simulink model "acev"  (R2020a)
settings: Solver=VariableStepAuto  StartTime=0.0  StopTime=10.0  RelTol=1e-3
undefined symbols (not defined in the file): DiscIntNeverNeededParam
libraries: simrfV2junction1 x11, powerlib x7, simulink x3, simrfV2elements x2, electricdrivelib x1, powerlib_meascontrol x1
settings Model: Creator=Asish Nayak  LastModifiedBy=Asish Nayak

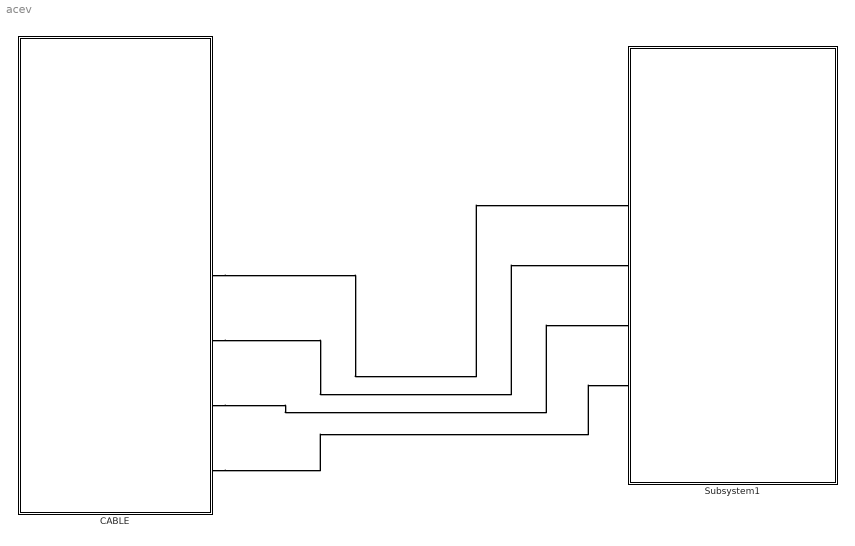
== system acev ==
  CABLE : Subsystem
  Subsystem1 : Subsystem
  connections:
  CABLE/RConn4 -- Subsystem1/LConn3
  CABLE/RConn5 -- Subsystem1/LConn4
  CABLE/RConn6 -- Subsystem1/LConn5
  CABLE/RConn7 -- Subsystem1/LConn6

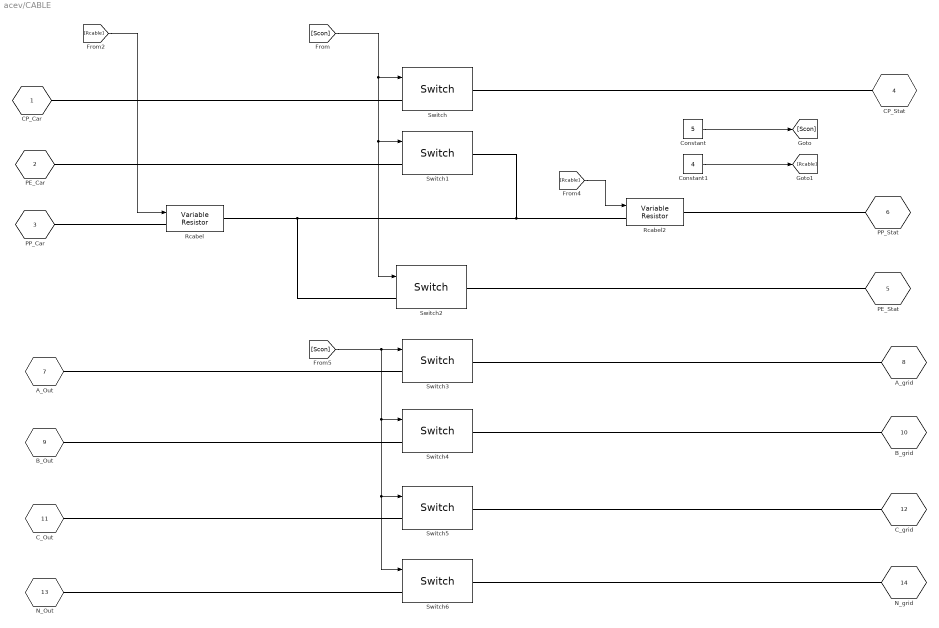
== system acev/CABLE ==
  Constant : Constant  Value=5
  Constant1 : Constant  Value=4
  Rcabel : simrfV2elements/Variable Resistor  classname=varresistor  hasNoise=on
      settings: SourceProductBaseCode=RB
  Rcabel2 : simrfV2elements/Variable Resistor  classname=varresistor  hasNoise=on
      settings: SourceProductBaseCode=RB
  Switch{,1..6} (7 alike) : simrfV2junction1/Switch  classname=switch  Ron=10 Ohm  Roff=1e6 Ohm  Vthres=0 V
      settings: SourceProductBaseCode=RB
  CP_Car : PMIOPort  Side=Left
  PE_Car : PMIOPort  Port=2  Side=Left
  PP_Car : PMIOPort  Port=3  Side=Left
  CP_Stat : PMIOPort  Port=4  Side=Right
  PE_Stat : PMIOPort  Port=5  Side=Right
  PP_Stat : PMIOPort  Port=6  Side=Right
  A_Out : PMIOPort  Port=7  Side=Left
  A_grid : PMIOPort  Port=8  Side=Right
  B_Out : PMIOPort  Port=9  Side=Left
  B_grid : PMIOPort  Port=10  Side=Right
  C_Out : PMIOPort  Port=11  Side=Left
  C_grid : PMIOPort  Port=12  Side=Right
  N_Out : PMIOPort  Port=13  Side=Left
  N_grid : PMIOPort  Port=14  Side=Right
  wires:
  Constant/1 -> [Scon]
  [Scon] -> Switch2/1, Switch1/1, Switch/1
  Constant1/1 -> [Rcable]
  [Rcable] -> Rcabel/1
  [Rcable] -> Rcabel2/1
  [Scon] -> Switch6/1, Switch5/1, Switch4/1, Switch3/1
  connections:
  CP_Car/RConn1 -- Switch/LConn1
  Switch1/LConn1 -- PE_Car/RConn1
  CP_Stat/RConn1 -- Switch/RConn1
  Rcabel/LConn1 -- PP_Car/RConn1
  Switch1/RConn1 -- Rcabel2/LConn1 -- Switch2/LConn1 -- Rcabel/RConn1
  PP_Stat/RConn1 -- Rcabel2/RConn1
  Switch2/RConn1 -- PE_Stat/RConn1
  N_Out/RConn1 -- Switch6/LConn1
  A_grid/RConn1 -- Switch3/RConn1
  C_Out/RConn1 -- Switch5/LConn1
  N_grid/RConn1 -- Switch6/RConn1
  C_grid/RConn1 -- Switch5/RConn1
  B_grid/RConn1 -- Switch4/RConn1
  A_Out/RConn1 -- Switch3/LConn1
  B_Out/RConn1 -- Switch4/LConn1

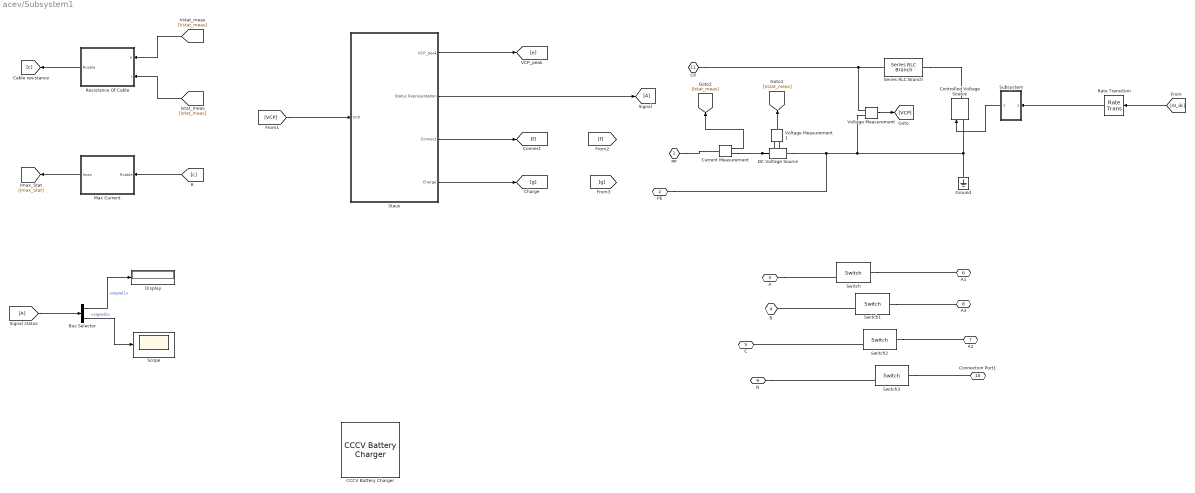
== system acev/Subsystem1 ==
  Bus Selector : BusSelector  OutputSignals=signal1,signal2
  CCCV Battery Charger : electricdrivelib/Extra Sources/CCCV Battery Charger  Preset=Custom specifications  P_nom=1500  s_type=3-phases AC (delta)  n_connect=off  eff_volt=208  in_freq=60  in_I_ripple=10  in_I_freq=1000  EFF_en=on  EFF_val=[0.627 0.803 0.855 0.871 0.872 0.864]  EFF_fu=[0.063 0.177 0.293 0.483 0.674 0.914]  THD_en=on  I_THD_val=[0.327 0.394 0.394 0.351 0.289 0.265]  I_THD_fu=[0.056 0.136 0.194 0.303 0.555 0.916]  H_DIST_rt=[0.199 1.297 0.328 0.029 0.416 0.200]  H_DIST_fr=[3 5 7 9 11 13]  PF_en=on  PF_val=[0.316 0.532 0.662 0.731 0.780 0.792]  PF_fu=[0.067 0.230 0.445 0.625 0.794 0.919]  Out_mode=Constant Current - Constant Voltage (CCCV)  DynInT=on  I_cst=10  V_cst=138  ABS_en=off  V_abs=142  ABS_end=Time based  ABS_time=3600  ABS_i=40  ripple=0.5  swF=1000  overshoot=1  stable_t=5  VoltComp=on  V_comp=-0.18  nom_temp=20
      settings: SourceProductBaseCode=PS
  Controlled Voltage Source : powerlib/Electrical Sources/Controlled Voltage Source  Initialize=off  Source_Type=DC  Amplitude=0  Phase=0  Frequency=0  Measurements=Voltage
  Current Measurement : powerlib/Measurements/Current Measurement  PhasorSimulation=off  OutputType=Complex  PSBequivalent=0
  DC Voltage Source : powerlib/Electrical Sources/DC Voltage Source  Amplitude=100  Measurements=None
  Display : Display
  Ground : powerlib/Elements/Ground  LConnTagsString=a
  Max Current : MATLAB Function  TreatAsAtomicUnit=on
  Rate Transition : RateTransition  InitialCondition=0.0  OutPortSampleTime=Tdc
  Resistance Of Cable : MATLAB Function  TreatAsAtomicUnit=on
  Scope : Scope
  Series RLC Branch : powerlib/Elements/Series RLC Branch  LConnTagsString=__new0  RConnTagsString=__new0  BranchType=R  Resistance=1000  Inductance=1e-3  SetiL0=off  InitialCurrent=0  Capacitance=1e-6  Setx0=off  InitialVoltage=0  Measurements=None
  Staus : Subsystem
  Subsystem : Subsystem
  Switch{,1..3} (4 alike) : simrfV2junction1/Switch  classname=switch  Ron=10 Ohm  Roff=1e6 Ohm  Vthres=0 V
      settings: SourceProductBaseCode=RB
  Voltage Measurement : powerlib/Measurements/Voltage Measurement  PhasorSimulation=off  OutputType=Complex  PSBequivalent=0
  Voltage Measurement1 : powerlib/Measurements/Voltage Measurement  PhasorSimulation=off  OutputType=Complex  PSBequivalent=0
  PP : PMIOPort  Side=Left
  PE : PMIOPort  Port=2  Side=Left
  A : PMIOPort  Port=3  Side=Left
  B : PMIOPort  Port=4  Side=Left
  C : PMIOPort  Port=5  Side=Left
  A1 : PMIOPort  Port=6  Side=Right
  A2 : PMIOPort  Port=7  Side=Right
  A3 : PMIOPort  Port=8  Side=Right
  N : PMIOPort  Port=9  Side=Left
  Connection Port1 : PMIOPort  Port=10  Side=Right
  CP : PMIOPort  Port=11  Side=Left
  wires:
  [SI_dc] -> Rate Transition/1
  Subsystem/1(Output) -> Controlled Voltage Source/1
  Rate Transition/1 -> Subsystem/1(Input)
  Voltage Measurement/1 -> [VCP]
  Voltage Measurement1/1 -> [Vstat_meas]
  Current Measurement/1 -> [Istat_meas]
  Bus Selector/2 -> Scope/1  "<signal2>"
  Bus Selector/1 -> Display/1  "<signal1>"
  Staus/4(Charge) -> [g]
  Staus/3(Connect) -> [f]
  Staus/1(VCP_peak) -> [e]
  [c] -> Max Current/1(Rcable)
  Staus/2(Status Representation) -> [A]
  Max Current/1(Imax) -> [Imax_Stat]
  [VCP] -> Staus/1(VCP)
  [A] -> Bus Selector/1
  [Istat_meas] -> Resistance Of Cable/2(I)
  Resistance Of Cable/1(Rcable) -> [c]
  [Vstat_meas] -> Resistance Of Cable/1(V)
  connections:
  Series RLC Branch/RConn1 -- Controlled Voltage Source/RConn1
  Voltage Measurement/LConn1 -- Series RLC Branch/LConn1 -- CP/RConn1
  Ground/LConn1 -- PE/RConn1 -- Voltage Measurement1/LConn2 -- DC Voltage Source/LConn1 -- Voltage Measurement/LConn2 -- Controlled Voltage Source/LConn1
  Current Measurement/RConn1 -- Voltage Measurement1/LConn1 -- DC Voltage Source/RConn1
  PP/RConn1 -- Current Measurement/LConn1
  A/RConn1 -- Switch/LConn1
  Switch/RConn1 -- A1/RConn1
  Switch1/LConn1 -- B/RConn1
  Switch1/RConn1 -- A3/RConn1
  Switch2/LConn1 -- C/RConn1
  Switch2/RConn1 -- A2/RConn1
  N/RConn1 -- Switch3/LConn1
  Switch3/RConn1 -- Connection Port1/RConn1

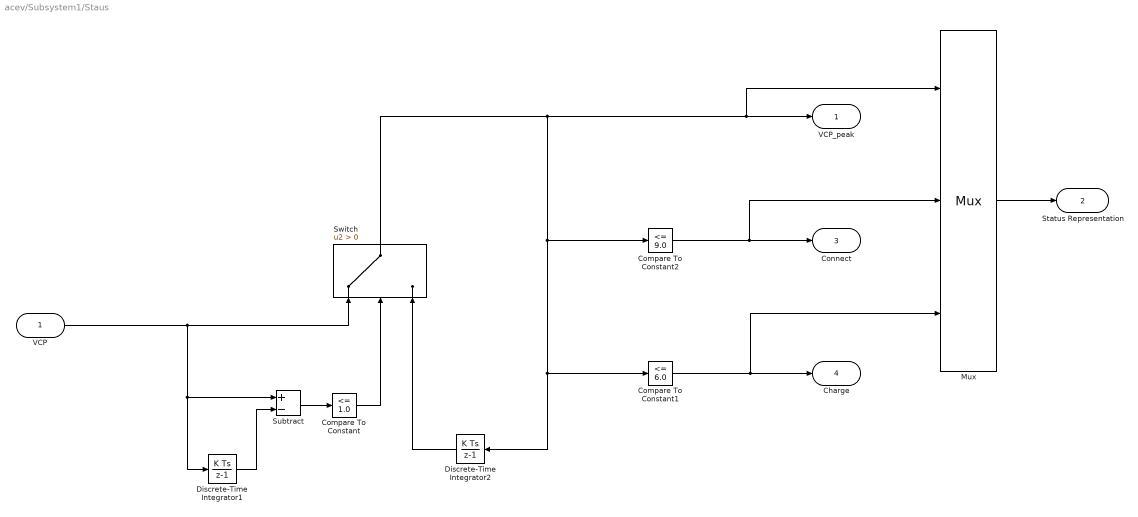
== system acev/Subsystem1/Staus ==
  VCP : Inport
  Compare To Constant : simulink/Logic and Bit Operations/Compare To Constant  relop=<=  const=1.0  OutDataTypeStr=boolean
  Compare To Constant1 : simulink/Logic and Bit Operations/Compare To Constant  relop=<=  const=6.0  OutDataTypeStr=boolean
  Compare To Constant2 : simulink/Logic and Bit Operations/Compare To Constant  relop=<=  const=9.0  OutDataTypeStr=boolean
  Discrete-Time Integrator1 : DiscreteIntegrator  SampleTime=-1  ICPrevOutput=DiscIntNeverNeededParam  ICPrevScaledInput=DiscIntNeverNeededParam
  Discrete-Time Integrator2 : DiscreteIntegrator  SampleTime=-1  ICPrevOutput=DiscIntNeverNeededParam  ICPrevScaledInput=DiscIntNeverNeededParam
  Mux : Mux  Inputs=3
      settings: DisplayOption=signals
  Subtract : Sum  Inputs=+-
  Switch : Switch  Criteria=u2 > Threshold
  VCP_peak : Outport  VectorParamsAs1DForOutWhenUnconnected=off
  Status Representation : Outport  Port=2  VectorParamsAs1DForOutWhenUnconnected=off
  Connect : Outport  Port=3  VectorParamsAs1DForOutWhenUnconnected=off
  Charge : Outport  Port=4  VectorParamsAs1DForOutWhenUnconnected=off
  wires:
  Switch/1 -> VCP_peak/1, Mux/1, Discrete-Time Integrator2/1, Compare To Constant1/1, Compare To Constant2/1
  Compare To Constant2/1 -> Connect/1, Mux/2
  VCP/1 -> Discrete-Time Integrator1/1, Subtract/1, Switch/1
  Subtract/1 -> Compare To Constant/1
  Discrete-Time Integrator2/1 -> Switch/3
  Discrete-Time Integrator1/1 -> Subtract/2
  Compare To Constant1/1 -> Charge/1, Mux/3
  Mux/1 -> Status Representation/1
  Compare To Constant/1 -> Switch/2

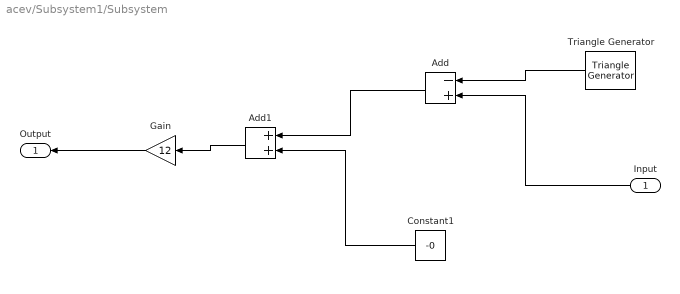
== system acev/Subsystem1/Subsystem ==
  Input : Inport
  Add : Sum  Inputs=-+
  Add1 : Sum
  Constant1 : Constant  Value=-0
  Gain : Gain  Gain=12
  Triangle Generator : powerlib_meascontrol/Pulse & Signal Generators/Triangle Generator  Freq=1e3  Phase=0  Ts=0
  Output : Outport
  wires:
  Triangle Generator/1 -> Add/1
  Input/1 -> Add/2
  Add/1 -> Add1/1
  Constant1/1 -> Add1/2
  Add1/1 -> Gain/1
  Gain/1 -> Output/1

== matlab function acev/Subsystem1/Resistance Of Cable ==
  data: V input; Rcable output; I input
function Rcable = fcn(V,I)
if( I< 0.0000001)
    Rcable=10000000;
    
else
    Rcable = V/I;

== matlab function acev/Subsystem1/Max Current ==
  data: Rcable input; Imax output
function Imax = fcn(Rcable)
if(Rcable<=101)
    Imax=63;
else if(Rcable<=221)
    Imax=32;
else if(Rcable<=681)
    Imax=20;
else if(Rcable<=1501)
    Imax=16;
else
    Imax=0;
